simulink model "CORDIC_divider"  (R2020b)
settings: Solver=VariableStepAuto  StartTime=0.0  StopTime=10.0  RelTol=1e-3
libraries: hdlsllib x2
settings Model: Creator=Luke  LastModifiedBy=Luke

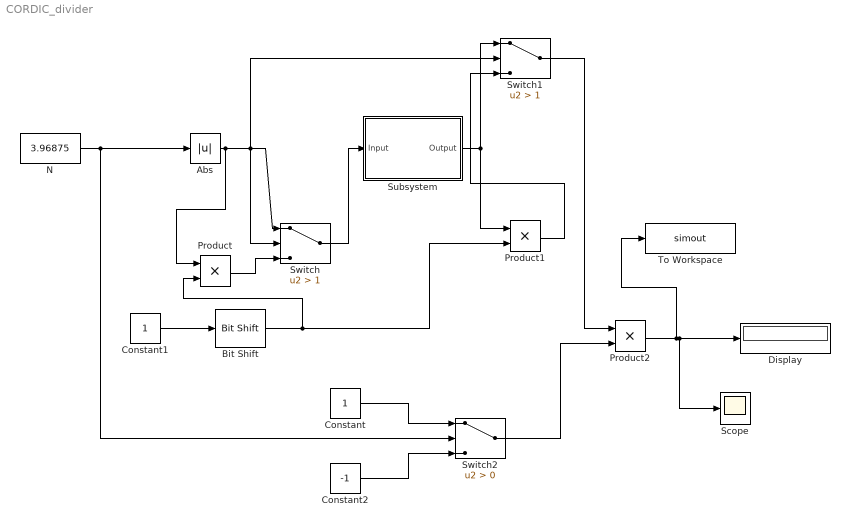
== system CORDIC_divider ==
  Abs : Abs
  Bit Shift : hdlsllib/Logic and Bit Operations/Bit Shift  mode=Shift Left Logical  N=5
  Constant : Constant
  Constant1 : Constant
  Constant2 : Constant  Value=-1
  Display : Display
  N : Constant  Value=3.96875
  Product : Product
  Product1 : Product
  Product2 : Product
  Scope : Scope
  Subsystem : Subsystem
  Switch : Switch  Criteria=u2 > Threshold  Threshold=1
  Switch1 : Switch  Criteria=u2 > Threshold  Threshold=1
  Switch2 : Switch  Criteria=u2 > Threshold
  To Workspace : ToWorkspace  VariableName=simout  SaveFormat=Timeseries  SampleTime=-1
  wires:
  N/1 -> Switch2/2, Abs/1
  Abs/1 -> Product/1, Switch1/2, Switch/2, Switch/1
  Constant1/1 -> Bit Shift/1
  Switch/1 -> Subsystem/1(Input)
  Bit Shift/1 -> Product1/2, Product/2
  Product/1 -> Switch/3
  Subsystem/1(Output) -> Product1/1, Switch1/1
  Product1/1 -> Switch1/3
  Switch1/1 -> Product2/1
  Constant/1 -> Switch2/1
  Constant2/1 -> Switch2/3
  Switch2/1 -> Product2/2
  Product2/1 -> To Workspace/1, Scope/1, Display/1

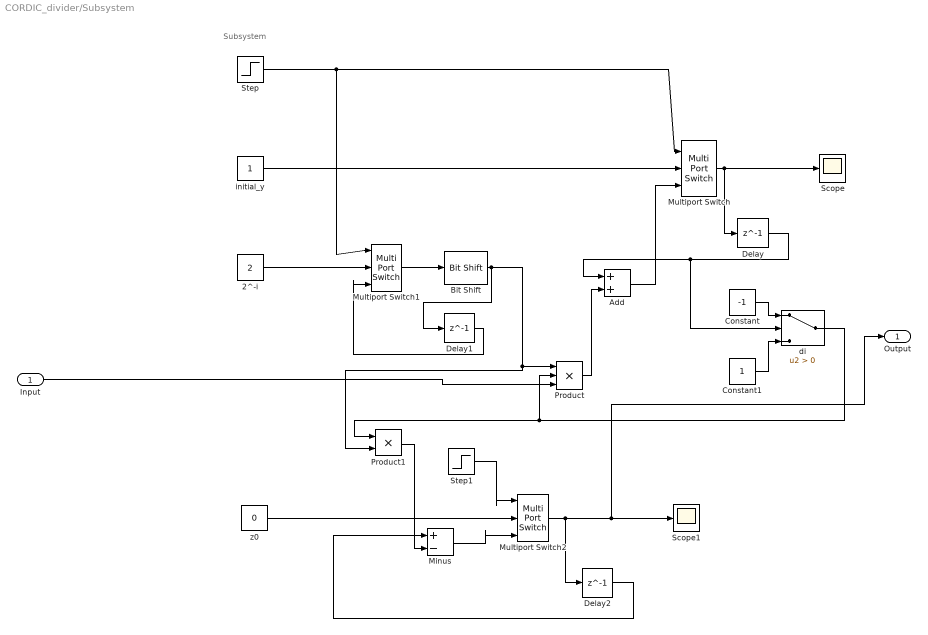
== system CORDIC_divider/Subsystem ==
  note: Subsystem
  Input : Inport
  2^-i : Constant  Value=2
  Add : Sum
  Bit Shift : hdlsllib/Logic and Bit Operations/Bit Shift  mode=Shift Right Arithmetic  N=1
  Constant : Constant  Value=-1
  Constant1 : Constant
  Delay : Delay  DelayLength=1
  Delay1 : Delay  DelayLength=1
  Delay2 : Delay  DelayLength=1
  Minus : Sum  Inputs=+-
  Multiport Switch : MultiPortSwitch  DataPortOrder=Zero-based contiguous  Inputs=2  zeroidx=on
  Multiport Switch1 : MultiPortSwitch  DataPortOrder=Zero-based contiguous  Inputs=2  zeroidx=on
  Multiport Switch2 : MultiPortSwitch  DataPortOrder=Zero-based contiguous  Inputs=2  zeroidx=on
  Product : Product  Inputs=3
  Product1 : Product
  Scope : Scope
  Scope1 : Scope
  Step : Step  SampleTime=0
  Step1 : Step  SampleTime=0
  di : Switch  Criteria=u2 > Threshold
  initial_y : Constant
  z0 : Constant  Value=0
  Output : Outport
  wires:
  Multiport Switch2/1 -> Output/1, Scope1/1, Delay2/1
  Input/1 -> Product/3
  Minus/1 -> Multiport Switch2/3
  initial_y/1 -> Multiport Switch/2
  Add/1 -> Multiport Switch/3
  Constant1/1 -> di/3
  Product1/1 -> Minus/2
  Multiport Switch1/1 -> Bit Shift/1
  Multiport Switch/1 -> Delay/1, Scope/1
  Product/1 -> Add/2
  Delay/1 -> di/2, Add/1
  2^-i/1 -> Multiport Switch1/2
  Step1/1 -> Multiport Switch2/1
  Delay1/1 -> Multiport Switch1/3
  Delay2/1 -> Minus/1
  Step/1 -> Multiport Switch1/1, Multiport Switch/1
  di/1 -> Product1/1, Product/2
  Constant/1 -> di/1
  z0/1 -> Multiport Switch2/2
  Bit Shift/1 -> Delay1/1, Product1/2, Product/1
